simulink model "SkywalkerX8_GuidanceAndNavigation_Verification"  (R2018a)
settings: Solver=FixedStepAuto  StartTime=0.0  StopTime=375  FixedStep=0.001  RelTol=1e-3
undefined symbols (not defined in the file): DiscIntNeverNeededParam, F, Light, magnitude, MIL, SkywalkerX8
libraries: simulink_extras x13, sensors x7, simulink x3, sharedTrackingLibrary x2, aerolibwind2 x1, dspmtrx3 x1, dspsigops x1
(part 3 of 3)

== system SkywalkerX8_GuidanceAndNavigation_Verification/State Estimation/Attitude Estimation Extended Kalman Filter with Filtering/Attitude Estimation Extended Kalman Filter ==
  u : Inport
  y : Inport  Port=2
  Attitude Estimation Extended Kalman Filter : sharedTrackingLibrary/Extended Kalman Filter  StateTransitionFcn=attitudeTransitionEstimate  HasStateTransitionJacobianFcn=on  StateTransitionJacobianFcn=attitudeTransitionEstimate_Jacobian  HasAdditiveProcessNoise=Additive  ProcessNoise=SkywalkerX8.Sensors.EKF.Attitude.ProcessCovarianceMatrix  HasTimeVaryingProcessNoise=off  HasStateTransitionFcnExtraArgument=1  InitialState=SkywalkerX8.Sensors.EKF.Attitude.InitialState  InitialStateCovariance=SkywalkerX8.Sensors.EKF.Attitude.InitialStateCovarianceMatrix  MeasurementFcn1=accelerometerMeasurementEstimate  HasMeasurementJacobianFcn1=on  MeasurementJacobianFcn1=accelerometerMeasurementEstimate_Jacobian  HasMeasurementEnablePort1=off  HasAdditiveMeasurementNoise1=Additive  MeasurementNoise1=SkywalkerX8.Sensors.EKF.Attitude.MeasurementCovarianceMatrix  HasTimeVaryingMeasurementNoise1=off  HasMeasurementFcnExtraArgument1=1  MeasurementFcn2=myMeasurementFcn  HasMeasurementJacobianFcn2=off  HasMeasurementEnablePort2=off  HasAdditiveMeasurementNoise2=Additive  MeasurementNoise2=1  HasTimeVaryingMeasurementNoise2=off  HasMeasurementFcnExtraArgument2=0  MeasurementFcn3=myMeasurementFcn  HasMeasurementJacobianFcn3=off  HasMeasurementEnablePort3=off  HasAdditiveMeasurementNoise3=Additive  MeasurementNoise3=1  HasTimeVaryingMeasurementNoise3=off  HasMeasurementFcnExtraArgument3=0  MeasurementFcn4=myMeasurementFcn  HasMeasurementJacobianFcn4=off  HasMeasurementEnablePort4=off  HasAdditiveMeasurementNoise4=Additive  MeasurementNoise4=1  HasTimeVaryingMeasurementNoise4=off  HasMeasurementFcnExtraArgument4=0  MeasurementFcn5=myMeasurementFcn  HasMeasurementJacobianFcn5=off  HasMeasurementEnablePort5=off  HasAdditiveMeasurementNoise5=Additive  MeasurementNoise5=1  HasTimeVaryingMeasurementNoise5=off  HasMeasurementFcnExtraArgument5=0  EnableMultirate=on  StateTransitionFcnSampleTime=SkywalkerX8.Sensors.EKF.Attitude.StateTransitionSampleTime  MeasurementFcn1SampleTime=SkywalkerX8.Sensors.EKF.Attitude.MeasurementSampleTime  MeasurementFcn2SampleTime=1  MeasurementFcn3SampleTime=1  MeasurementFcn4SampleTime=1  MeasurementFcn5SampleTime=1  UseCurrentEstimator=on  OutputStateCovariance=off  DataType=double  SampleTime=SkywalkerX8.Sensors.EKF.Attitude.StateTransitionSampleTime  NumberOfMeasurements=1
      settings: SourceProductName=Control System Toolbox  SourceProductBaseCode=CT
  Constant : Constant  Value=SkywalkerX8.Sensors.EKF.Attitude.StateTransitionSampleTime
  Mux : Mux  Inputs=2
  Rate Transition : RateTransition  InitialCondition=SkywalkerX8.Sensors.EKF.Attitude.InitialInput  OutPortSampleTime=SkywalkerX8.Sensors.EKF.Attitude.StateTransitionSampleTime
  Rate Transition1 : RateTransition  InitialCondition=SkywalkerX8.Sensors.EKF.Attitude.InitialInput  OutPortSampleTime=SkywalkerX8.Sensors.EKF.Attitude.MeasurementSampleTime
  Rate Transition2 : RateTransition  InitialCondition=SkywalkerX8.Sensors.EKF.Attitude.InitialMeasurement  OutPortSampleTime=SkywalkerX8.Sensors.EKF.Attitude.MeasurementSampleTime
  xhat : Outport
  wires:
  y/1 -> Rate Transition2/1
  u/1 -> Rate Transition1/1, Rate Transition/1
  Attitude Estimation Extended Kalman Filter/1 -> xhat/1
  Rate Transition1/1 -> Attitude Estimation Extended Kalman Filter/3
  Rate Transition2/1 -> Attitude Estimation Extended Kalman Filter/2
  Mux/1 -> Attitude Estimation Extended Kalman Filter/1
  Rate Transition/1 -> Mux/1
  Constant/1 -> Mux/2

== system SkywalkerX8_GuidanceAndNavigation_Verification/Autopilot Digital/Gain Scheduled Controller Chi Digital/PIDF Controller Va_theta/Clamping circuit ==
  preSat : Inport  DisableCoverage=on
  postSat : Inport  DisableCoverage=on  Port=2
  Memory : Memory  DisableCoverage=on
  NotEqual : RelationalOperator  DisableCoverage=on  Operator=~=  RndMeth=Nearest  InputSameDT=on
  Clamp : Outport  DisableCoverage=on
  wires:
  postSat/1 -> NotEqual/2
  preSat/1 -> NotEqual/1
  NotEqual/1 -> Memory/1
  Memory/1 -> Clamp/1

== system SkywalkerX8_GuidanceAndNavigation_Verification/Autopilot Digital/Gain Scheduled Controller Phi Digital/PI Controller Phi/Clamping circuit ==
  preSat : Inport  DisableCoverage=on
  postSat : Inport  DisableCoverage=on  Port=2
  Memory : Memory  DisableCoverage=on
  NotEqual : RelationalOperator  DisableCoverage=on  Operator=~=  RndMeth=Nearest  InputSameDT=on
  Clamp : Outport  DisableCoverage=on
  wires:
  postSat/1 -> NotEqual/2
  preSat/1 -> NotEqual/1
  NotEqual/1 -> Memory/1
  Memory/1 -> Clamp/1

== system SkywalkerX8_GuidanceAndNavigation_Verification/Autopilot Digital/Gain Scheduled Controller Theta Digital/PI Controller Theta/Clamping circuit ==
  preSat : Inport  DisableCoverage=on
  postSat : Inport  DisableCoverage=on  Port=2
  Memory : Memory  DisableCoverage=on
  NotEqual : RelationalOperator  DisableCoverage=on  Operator=~=  RndMeth=Nearest  InputSameDT=on
  Clamp : Outport  DisableCoverage=on
  wires:
  postSat/1 -> NotEqual/2
  preSat/1 -> NotEqual/1
  NotEqual/1 -> Memory/1
  Memory/1 -> Clamp/1

== system SkywalkerX8_GuidanceAndNavigation_Verification/Autopilot Digital/Gain Scheduled Controller Va_dt Digital/PIDF Controller Va_dt/Clamping circuit ==
  preSat : Inport  DisableCoverage=on
  postSat : Inport  DisableCoverage=on  Port=2
  Memory : Memory  DisableCoverage=on
  NotEqual : RelationalOperator  DisableCoverage=on  Operator=~=  RndMeth=Nearest  InputSameDT=on
  Clamp : Outport  DisableCoverage=on
  wires:
  postSat/1 -> NotEqual/2
  preSat/1 -> NotEqual/1
  NotEqual/1 -> Memory/1
  Memory/1 -> Clamp/1

== system SkywalkerX8_GuidanceAndNavigation_Verification/Autopilot Digital/Gain Scheduled Controller Va_theta Digital/PIDF Controller Va_theta/Clamping circuit ==
  preSat : Inport  DisableCoverage=on
  postSat : Inport  DisableCoverage=on  Port=2
  Memory : Memory  DisableCoverage=on
  NotEqual : RelationalOperator  DisableCoverage=on  Operator=~=  RndMeth=Nearest  InputSameDT=on
  Clamp : Outport  DisableCoverage=on
  wires:
  postSat/1 -> NotEqual/2
  preSat/1 -> NotEqual/1
  NotEqual/1 -> Memory/1
  Memory/1 -> Clamp/1

== system SkywalkerX8_GuidanceAndNavigation_Verification/Autopilot Digital/Gain Scheduled Controller h_theta Digital/PIDF Controller h_theta/Clamping circuit ==
  preSat : Inport  DisableCoverage=on
  postSat : Inport  DisableCoverage=on  Port=2
  Memory : Memory  DisableCoverage=on
  NotEqual : RelationalOperator  DisableCoverage=on  Operator=~=  RndMeth=Nearest  InputSameDT=on
  Clamp : Outport  DisableCoverage=on
  wires:
  postSat/1 -> NotEqual/2
  preSat/1 -> NotEqual/1
  NotEqual/1 -> Memory/1
  Memory/1 -> Clamp/1

== matlab function SkywalkerX8_GuidanceAndNavigation_Verification/Guidance and Navigation/Path Following Algorithm/Orbit Following ==
  data: c input size=3, 1; h_c output; rho input; lambda input; p input size=3, 1; chi input; chi_c output; korbit parameter
function [h_c, chi_c] = fcn(c, rho, lambda, p, chi, korbit)

    [h_c, chi_c] = orbitFollowing(c, rho, lambda, p, chi, korbit);

end

== matlab function SkywalkerX8_GuidanceAndNavigation_Verification/SkywalkerX8 Aircraft + Aerodynamics Observable Feedback/Rotatation Vehicle to Body ==
  data: PhiThetaPsi input; uwvwww output; wnwewd input
function uwvwww = fcn(PhiThetaPsi, wnwewd)

    Phi = PhiThetaPsi(1);
    Theta = PhiThetaPsi(2);
    Psi = PhiThetaPsi(3);

    Rvb = [cos(Theta)*cos(Psi)                             , cos(Theta)*sin(Psi)                             , -sin(Theta)        ;
           sin(Phi)*sin(Theta)*cos(Psi) - cos(Phi)*sin(Psi), sin(Phi)*sin(Theta)*sin(Psi) + cos(Phi)*cos(Psi), sin(Phi)*cos(Theta);
           cos(Phi)*sin(Theta)*cos(Psi) + sin(Phi)*sin(Psi), cos(Phi)*sin(Theta)*sin(Psi) - sin(Phi)*cos(Psi), cos(Phi)*cos(Theta)];

    wnwewed = reshape(wnwewd, 3, 1);

    uwvwww = Rvb*wnwewed;
    
end

== stateflow chart SkywalkerX8_GuidanceAndNavigation_Verification/Autopilot Digital/Altitude Control State Machine ==
  settings: executeAtInitialization=1
  state Descend_Zone
    during: dt = 0
    during: theta_c = theta_c_Va
  state Altitude_Hold_Zone
    during: dt = dt_Va
    during: theta_c = theta_c_h
  state Landing_Mode
    during: dt = 0
    during: theta_c = theta_c_h
  state Climb_Zone
    during: dt = 1.0
    during: theta_c = theta_c_Va
  state Take_Off_Zone
    during: dt = 1.0
    during: theta_c = theta_c_takeoff
  state Pre_Flight
    during: dt = dt_Va
    during: theta_c = theta_c_h
  Descend_Zone -> Landing_Mode [order 2] : [ h_c == 0 ]
  Altitude_Hold_Zone -> Descend_Zone [order 2] : [h >= (h_c + h_hold*(1+hyst_frac))]
  Descend_Zone -> Altitude_Hold_Zone [order 1] : [h < (h_c + h_hold*(1-hyst_frac))]
  Altitude_Hold_Zone -> Landing_Mode [order 3] : [ h_c == 0 ]
  Pre_Flight -> Altitude_Hold_Zone [order 1] : [PreFlightBypass]
  Climb_Zone -> Altitude_Hold_Zone [order 2] : [h >= (h_c - h_hold*(1+hyst_frac))]
  Altitude_Hold_Zone -> Climb_Zone [order 1] : [h < (h_c - h_hold*(1-hyst_frac))]
  Climb_Zone -> Landing_Mode [order 3] : [ h_c == 0 ]
  Take_Off_Zone -> Landing_Mode [order 2] : [ h_c == 0 ]
  Landing_Mode -> Pre_Flight : [ h == 0 ]
  Take_Off_Zone -> Climb_Zone [order 1] : [h >= h_takeoff*(1+hyst_frac)]
  Climb_Zone -> Take_Off_Zone [order 1] : [h < h_takeoff*(1-hyst_frac)]
  Pre_Flight -> Take_Off_Zone [order 2] : [ h_c > 0 ]
  (default) -> Pre_Flight
  data: dt_Va input; theta_c_Va input; theta_c_h input; h input; h_c input; dt output; theta_c output; h_hold parameter double; theta_c_takeoff parameter double; h_takeoff parameter double; hyst_frac parameter double; PreFlightBypass parameter

== matlab function SkywalkerX8_GuidanceAndNavigation_Verification/State Estimation/GPS Smoothing Extended Kalman Filter/Reciprocal ==
  data: u input; y output
function y = reciprocal(u)

    if (u ~= 0)
       y = 1/u;
    else
       y = 1E06; 
    end

end

== matlab function SkywalkerX8_GuidanceAndNavigation_Verification/Guidance and Navigation/Path Following Algorithm/Straight Line Path Following ==
  data: r input size=3, 1; h_c output; chi_c output; q input size=3, 1; p input size=3, 1; chi input size=1; chi_inf parameter; kpath parameter
function [h_c, chi_c] = fcn(r, q, p, chi, chi_inf, kpath)

    [h_c, chi_c] = straightLineFollowing(r, q, p, chi, chi_inf, kpath);

end

== matlab function SkywalkerX8_GuidanceAndNavigation_Verification/Guidance and Navigation/Fillet Path Manager/Path Manager Follow Waypoints Fillet ==
  data: r output size=3, 1; q output size=3, 1; c output size=3, 1; rho output size=1; lambda output size=1; W input; WChangeCheck input; flag output size=1; p input size=3, 1; R input; prev_state input; prev_i input; i output size=1
function [r, q, c, rho, lambda, flag, i] = fcn(W, WChangeCheck, p, R, prev_state, prev_i)
    
    [r, q, c, rho, lambda, flag, i] = pathManager_followWaypointsFillet(W, WChangeCheck, p, R, prev_state, prev_i);

end

== matlab function SkywalkerX8_GuidanceAndNavigation_Verification/Guidance and Navigation/Banked Turn Turn Radius Calculation ==
  data: Vg input; R output; theta input; alpha input; g parameter; phi_max parameter; SF parameter
function R = turnRadius(Vg, theta, alpha, g, phi_max, SF)
    
    % Minimum turn radius assuming no wind or sideslip

    gamma = theta - alpha;
    
    % We use 0.5 of the maximum roll angle as we need to roll to the max and
    % then back to 0, so assume that we're at 0.5 of that equivalently.
    
    R = SF*(Vg^2)*cos(gamma)/( g*tan(0.5*phi_max) );
    
end

== matlab function SkywalkerX8_GuidanceAndNavigation_Verification/State Estimation/GPS Smoothing Extended Kalman Filter/MATLAB Function ==
  data: chi input; chi_wrap output
function chi_wrap = wrap(chi)

    chi_wrap = chi;

    while chi_wrap < -pi
       chi_wrap = chi_wrap + 2*pi; 
    end

    while chi_wrap > pi
       chi_wrap = chi_wrap - 2*pi; 
    end

end
